simulink model "minimalIpCore"  (R2024a)
settings: Solver=FixedStepDiscrete  StartTime=0.0  StopTime=stopTime  RelTol=1e-3
values from neighbouring files (symbols this model uses):
  fs = 100e6    (= 100000000)    [testMinimalIpCore.m]
libraries: dspsrcs4 x2
settings Model: DataTypeOverride=Off  Creator=cotti  LastModifiedBy=cotti
settings OptimizationCC: BlockReduction=off  ConditionallyExecuteInputs=off  DefaultParameterBehavior=Inlined  InheritOutputTypeSmallerThanSingle=on
settings DebuggingCC: AlgebraicLoopMsg=error  SingleTaskRateTransMsg=error  UnconnectedInputMsg=warning  UnconnectedOutputMsg=warning  UnconnectedLineMsg=warning
settings HardwareCC: ProdBitPerPointer=32  ProdBitPerSizeT=32  ProdBitPerPtrDiffT=32  ProdLargestAtomicFloat=None  ProdIntDivRoundTo=Undefined  ProdEndianess=Unspecified  ProdWordSize=32  ProdHWDeviceType=ASIC/FPGA->ASIC/FPGA  TargetBitPerLong=64  TargetBitPerPointer=64  TargetBitPerSizeT=64  TargetBitPerPtrDiffT=64  TargetLongLongMode=on  TargetIntDivRoundTo=Zero  TargetEndianess=LittleEndian  TargetWordSize=64  TargetHWDeviceType=Custom Processor->MATLAB Host Computer  ProdEqTarget=off

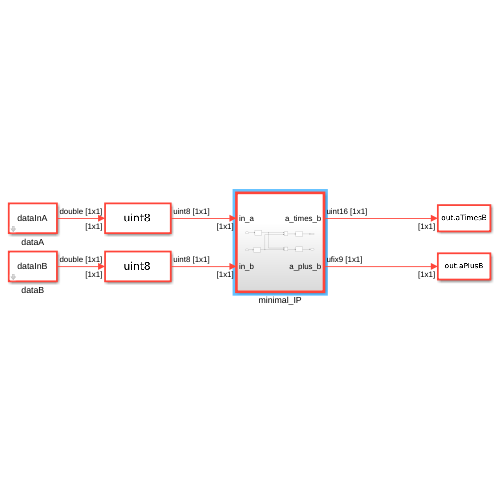
[thumbnail: Simulink's stored preview of the top-level diagram]
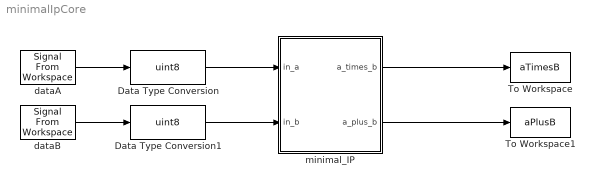
== system minimalIpCore ==
  Data Type Conversion : DataTypeConversion  OutDataTypeStr=uint8  SaturateOnIntegerOverflow=off  RndMeth=Floor
  Data Type Conversion1 : DataTypeConversion  OutDataTypeStr=uint8  SaturateOnIntegerOverflow=off  RndMeth=Floor
  To Workspace : ToWorkspace  VariableName=aTimesB  SampleTime=1/fs
      settings: Save2DSignal=2-D array (concatenate along first dimension)
  To Workspace1 : ToWorkspace  VariableName=aPlusB  SampleTime=1/fs
      settings: Save2DSignal=2-D array (concatenate along first dimension)
  dataA : dspsrcs4/Signal From Workspace  X=dataInA  Ts=1/fs  nsamps=1  OutputAfterFinalValue=Setting to zero  ignoreOrWarnInputAndFrameLengths=off  OutputFrames=off
  dataB : dspsrcs4/Signal From Workspace  X=dataInB  Ts=1/fs  nsamps=1  OutputAfterFinalValue=Setting to zero  ignoreOrWarnInputAndFrameLengths=off  OutputFrames=off
  minimal_IP : Subsystem  TreatAsAtomicUnit=on
  wires:
  dataA/1 -> Data Type Conversion/1
  minimal_IP/1(a_times_b) -> To Workspace/1
  minimal_IP/2(a_plus_b) -> To Workspace1/1
  dataB/1 -> Data Type Conversion1/1
  Data Type Conversion/1 -> minimal_IP/1(in_a)
  Data Type Conversion1/1 -> minimal_IP/2(in_b)

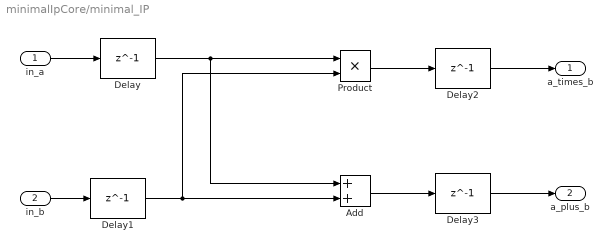
== system minimalIpCore/minimal_IP ==
  in_a : Inport
  in_b : Inport  Port=2
  Add : Sum
  Delay{,1..3} (4 alike) : Delay  DelayLength=1  InitialCondition=0  UseCircularBuffer=on
  Product : Product
  a_times_b : Outport
  a_plus_b : Outport  Port=2
  wires:
  in_a/1 -> Delay/1
  in_b/1 -> Delay1/1
  Product/1 -> Delay2/1
  Delay2/1 -> a_times_b/1
  Delay3/1 -> a_plus_b/1
  Add/1 -> Delay3/1
  Delay/1 -> Add/1, Product/1
  Delay1/1 -> Product/2, Add/2
